simulink model "AOOstateflow"  (R2022a)
settings: Solver=FixedStepAuto  StartTime=0.0  StopTime=100.0  FixedStep=1e-3  RelTol=1e-3  EnableMultiTasking=on
undefined symbols (not defined in the file): D10, D11, D12, D2, D3, D8, D9, PTA0, PTA1, PTB9, PTC4, PTD0, PTD2, PTD3
libraries: frdmk64flib x7
settings Model: ExtModeTrigDuration=5  Creator=sabri  LastModifiedBy=Potat
settings SolverCC: AlgebraicLoopSolver=TrustRegion
settings OptimizationCC: EnhancedBackFolding=on  PassReuseOutputArgsAs=Individual arguments  ZeroExternalMemoryAtStartup=off  ZeroInternalMemoryAtStartup=off  MaxStackSize=64  OptimizeBlockOrder=speed  DifferentSizesBufferReuse=on  OptimizationCustomize=off  EfficientTunableParamExpr=on
settings DebuggingCC: ParameterTunabilityLossMsg=error  UnconnectedInputMsg=warning  UnconnectedOutputMsg=warning  UnconnectedLineMsg=warning  SFMachineParentedDataDiag=warning
settings HardwareCC: ProdBitPerPointer=32  ProdBitPerSizeT=32  ProdBitPerPtrDiffT=32  ProdLargestAtomicInteger=Long  ProdLargestAtomicFloat=Double  ProdWordSize=32  ProdHWDeviceType=ARM Compatible->ARM Cortex
settings SFSimCC: MATLABDynamicMemAlloc=off
settings RTWCC: SystemTargetFile=ert.tlc  HardwareBoard=NXP FRDM-K64F  TLCOptions="-aInlineSetEventsForThisBaseRateFcn=TLC_FALSE -aSuppressMultiTaskScheduler=TLC_FALSE  -aRateBasedStepFcn=0"  TemplateMakefile=ert_default_tmf  Toolchain=GNU Tools for ARM Embedded Processors
settings CodeAppCC: ForceParamTrailComments=on  IgnoreCustomStorageClasses=off  OperatorAnnotations=on  SimulinkDataObjDesc=on  SFDataObjDesc=on  InsertBlockDesc=on

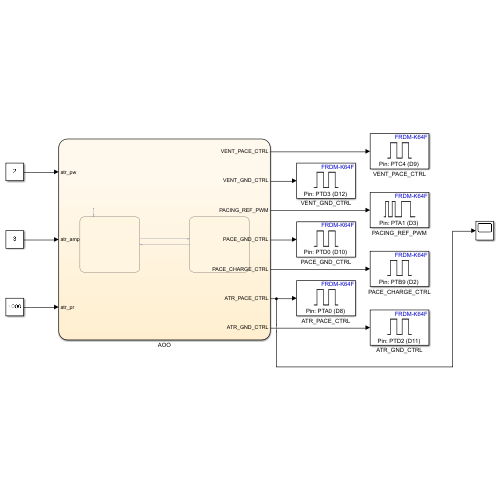
[thumbnail: Simulink's stored preview of the top-level diagram]
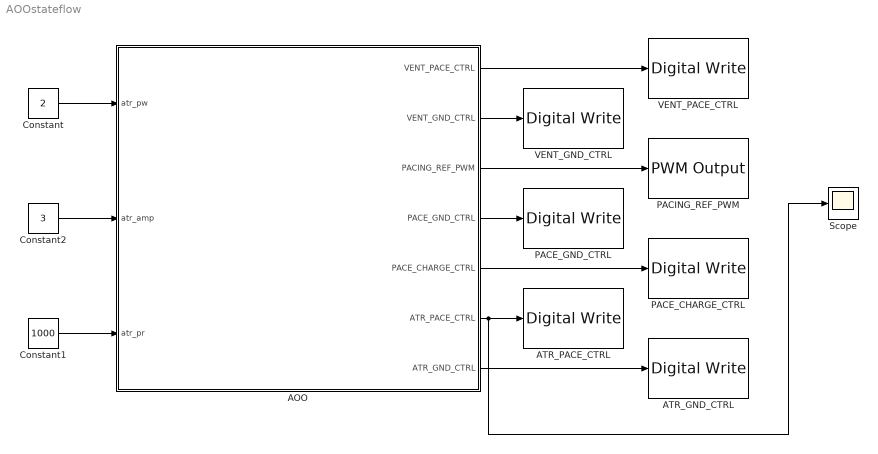
== system AOOstateflow ==
  AOO : Stateflow chart  TreatAsAtomicUnit=on
  ATR_GND_CTRL : frdmk64flib/Digital Write  Whichpin=PTD2 (D11)
  ATR_PACE_CTRL : frdmk64flib/Digital Write  Whichpin=PTA0 (D8)
  Constant : Constant  Value=2
  Constant1 : Constant  Value=1000
  Constant2 : Constant  Value=3
  PACE_CHARGE_CTRL : frdmk64flib/Digital Write  Whichpin=PTB9 (D2)
  PACE_GND_CTRL : frdmk64flib/Digital Write  Whichpin=PTD0 (D10)
  PACING_REF_PWM : frdmk64flib/PWM Output  Whichpin=PTA1 (D3)  InitialFrequency=2000  InitialDutyCycle=0
  Scope : Scope
  VENT_GND_CTRL : frdmk64flib/Digital Write  Whichpin=PTD3 (D12)
  VENT_PACE_CTRL : frdmk64flib/Digital Write  Whichpin=PTC4 (D9)
  wires:
  Constant/1 -> AOO/1(atr_pw)
  Constant1/1 -> AOO/3(atr_pr)
  Constant2/1 -> AOO/2(atr_amp)
  AOO/5(PACE_CHARGE_CTRL) -> PACE_CHARGE_CTRL/1
  AOO/4(PACE_GND_CTRL) -> PACE_GND_CTRL/1
  AOO/2(VENT_GND_CTRL) -> VENT_GND_CTRL/1
  AOO/1(VENT_PACE_CTRL) -> VENT_PACE_CTRL/1
  AOO/3(PACING_REF_PWM) -> PACING_REF_PWM/1
  AOO/6(ATR_PACE_CTRL) -> Scope/1, ATR_PACE_CTRL/1
  AOO/7(ATR_GND_CTRL) -> ATR_GND_CTRL/1

== stateflow chart AOOstateflow/AOO ==
  state Charging_Heart
    entry:
    PACE_CHARGE_CTRL = 0
    VENT_PACE_CTRL = 0
    ATR_PACE_CTRL = 1
    VENT_GND_CTRL = 0
    ATR_GND_CTRL = 0
    PACE_GND_CTRL = 1
    PACING_REF_PWM = atr_amp/5*100
  state Discharging_Heart
    entry:
    PACE_CHARGE_CTRL = 1
    VENT_PACE_CTRL = 0
    ATR_PACE_CTRL = 0
    VENT_GND_CTRL = 0
    ATR_GND_CTRL = 1
    PACE_GND_CTRL = 1
  (default) -> Charging_Heart
  Charging_Heart -> Discharging_Heart : [after(atr_pw, msec)]
  Discharging_Heart -> Charging_Heart : [after(atr_pr - atr_pw, msec)]
  data: atr_pw input; atr_amp input; atr_pr input; VENT_PACE_CTRL output; VENT_GND_CTRL output; PACING_REF_PWM output; PACE_GND_CTRL output; PACE_CHARGE_CTRL output; ATR_PACE_CTRL output; ATR_GND_CTRL output
